simulink model "unforcedPendulum"  (R2025a)
settings: Solver=VariableStepAuto  StartTime=0.0  StopTime=10.0  RelTol=1e-3
model workspace (MAT data in the model file):
  M = 0.5
  Ts = 0.01
  b = 0.1
  g = 9.8
  l = 0.5
  m = 0.2
settings Model: Creator=JPIRES3  LastModifiedBy=JPIRES3

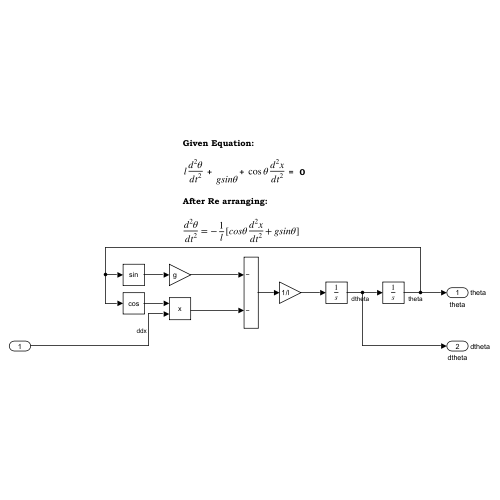
[thumbnail: Simulink's stored preview of the top-level diagram]
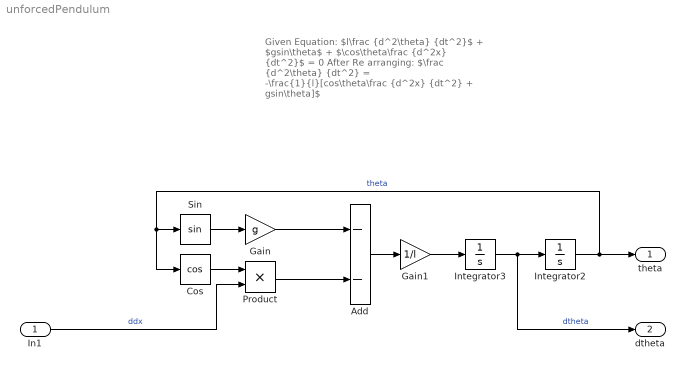
== system unforcedPendulum ==
  note: Given Equation:
      |
      | $l\frac {d^2\theta} {dt^2}$ + $gsin\theta$ + $\cos\theta\frac {d^2x} {dt^2}$ = 0
      |
      | After Re arranging:
      |
      | $\frac {d^2\theta} {dt^2} = -\frac{1}{l}[cos\theta\frac {d^2x} {dt^2} + gsin\theta]$
  In1 : Inport
  Add : Sum  Inputs=--
  Cos : Trigonometry  Operator=cos
  Gain : Gain  Gain=g
  Gain1 : Gain  Gain=1/l
  Integrator2 : Integrator  InitialCondition=0.9*pi
  Integrator3 : Integrator  InitialCondition=0.9*pi
  Product : Product
  Sin : Trigonometry
  theta : Outport  SignalName=theta
  dtheta : Outport  Port=2  SignalName=dtheta
  wires:
  In1/1 -> Product/2  "ddx"
  Integrator3/1 -> dtheta/1, Integrator2/1  "dtheta"
  Gain/1 -> Add/1
  Product/1 -> Add/2
  Add/1 -> Gain1/1
  Integrator2/1 -> theta/1, Cos/1, Sin/1  "theta"
  Sin/1 -> Gain/1
  Cos/1 -> Product/1
  Gain1/1 -> Integrator3/1
